simulink model "dummy"  (R2020a)
settings: Solver=VariableStepAuto  StartTime=0.0  StopTime=inf  RelTol=1e-3
undefined symbols (not defined in the file or in its folder): gain_l, num_l, wn_l, Z0_l, Z1_l, Z2_l, zeta_l
libraries: robotlib x1
settings Model: EnablePacing=on  Creator=lamarre  LastModifiedBy=lamarre

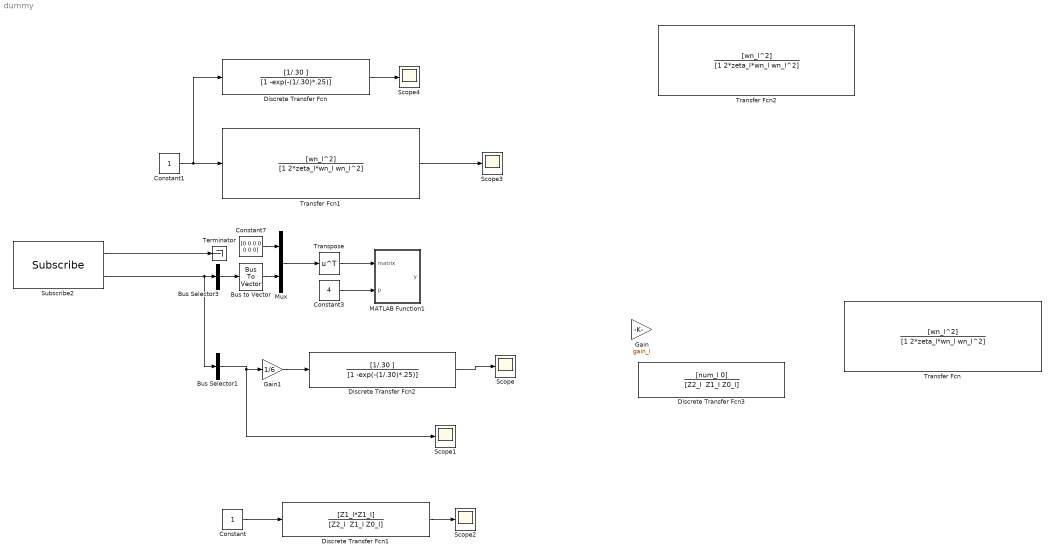
== system dummy ==
  Bus Selector1 : BusSelector  OutputSignals=Linear.X  OutputAsBus=on
  Bus Selector3 : BusSelector  OutputSignals=Linear.X,Linear.Y,Linear.Z,Angular.X,Angular.Y,Angular.Z  OutputAsBus=on
  Bus to Vector : BusToVector
  Constant : Constant
  Constant1 : Constant
  Constant3 : Constant  Value=4
  Constant7 : Constant  Value=[0 0 0 0 0 0 0]
  Discrete Transfer Fcn : DiscreteTransferFcn  Numerator=[1/.30 ]  Denominator=[1 -exp(-(1/.30)*.25)]  SampleTime=.25
  Discrete Transfer Fcn1 : DiscreteTransferFcn  Numerator=[Z1_l*Z1_l]  Denominator="[Z2_l  Z1_l Z0_l]"  SampleTime=1/4
  Discrete Transfer Fcn2 : DiscreteTransferFcn  Numerator=[1/.30 ]  Denominator=[1 -exp(-(1/.30)*.25)]  SampleTime=.25
  Discrete Transfer Fcn3 : DiscreteTransferFcn  Numerator=[num_l 0]  Denominator="[Z2_l  Z1_l Z0_l]"  SampleTime=1/4
  Gain : Gain  Gain=gain_l
  Gain1 : Gain  Gain=1/6
  MATLAB Function1 : MATLAB Function  TreatAsAtomicUnit=on
  Mux : Mux  Inputs=2
  Scope{,1..4} (5 alike) : Scope
  Subscribe2 : robotlib/Subscribe  topicSource=Specify your own  topic=/spacenav/twist  messageType=geometry_msgs/Twist  sampleTime=1/30  messageQueueLength=2
  Terminator : Terminator
  Transfer Fcn : TransferFcn  Numerator=[wn_l^2]  Denominator=[1 2*zeta_l*wn_l wn_l^2]
  Transfer Fcn1 : TransferFcn  Numerator=[wn_l^2]  Denominator=[1 2*zeta_l*wn_l wn_l^2]
  Transfer Fcn2 : TransferFcn  Numerator=[wn_l^2]  Denominator=[1 2*zeta_l*wn_l wn_l^2]
  Transpose : Math  Operator=transpose  SaturateOnIntegerOverflow=on
  wires:
  Constant3/1 -> MATLAB Function1/2(p)
  Mux/1 -> Transpose/1
  Bus Selector3/1 -> Bus to Vector/1
  Subscribe2/1 -> Terminator/1
  Constant7/1 -> Mux/1
  Bus to Vector/1 -> Mux/2
  Subscribe2/2 -> Bus Selector1/1, Bus Selector3/1
  Transpose/1 -> MATLAB Function1/1(matrix)
  Constant/1 -> Discrete Transfer Fcn1/1
  Discrete Transfer Fcn1/1 -> Scope2/1
  Constant1/1 -> Discrete Transfer Fcn/1, Transfer Fcn1/1
  Transfer Fcn1/1 -> Scope3/1
  Discrete Transfer Fcn2/1 -> Scope/1
  Discrete Transfer Fcn/1 -> Scope4/1
  Gain1/1 -> Discrete Transfer Fcn2/1
  Bus Selector1/1 -> Gain1/1, Scope1/1

== matlab function dummy/MATLAB Function1 ==
  data: matrix input; y output size=[4 13]; p input
function y = fcn(matrix,p)
matrix(10)=-matrix(10);
y = repmat(matrix,4,1);
